simulink model "Copy_of_model_test"  (R2018b)
settings: Solver=ode5  StartTime=0.0  StopTime=10.0  FixedStep=0.01  RelTol=1e-3
values from neighbouring files (symbols this model uses):
  g = 9.81    [equations.m]    (also in general.m; general_lqi.m)
  m = 0.06    [equations.m]    (also in general.m = 0.057; general_lqi.m = 0.057)
  R = 1    [evaluateL.m]    (also in general.m = 4; general_lqi.m = 4)
  u_0 = R*x3_0    [general.m]    (also in general_lqi.m)
  x1_0 = 0.005    [general.m]    (also in general_lqi.m = 0.01)
  x2_0 = 0    [general.m]    (also in general_lqi.m)
  x3_0 = sqrt((-2*m*g)/first(x1_0))    [general.m]    (also in general_lqi.m)
  x_0 = [x1_0 x2_0 x3_0]    [general.m]    (also in general_lqi.m)
undefined symbols (not defined in the file or in its folder): K
settings Model: Creator=Kinga  LastModifiedBy=Kinga

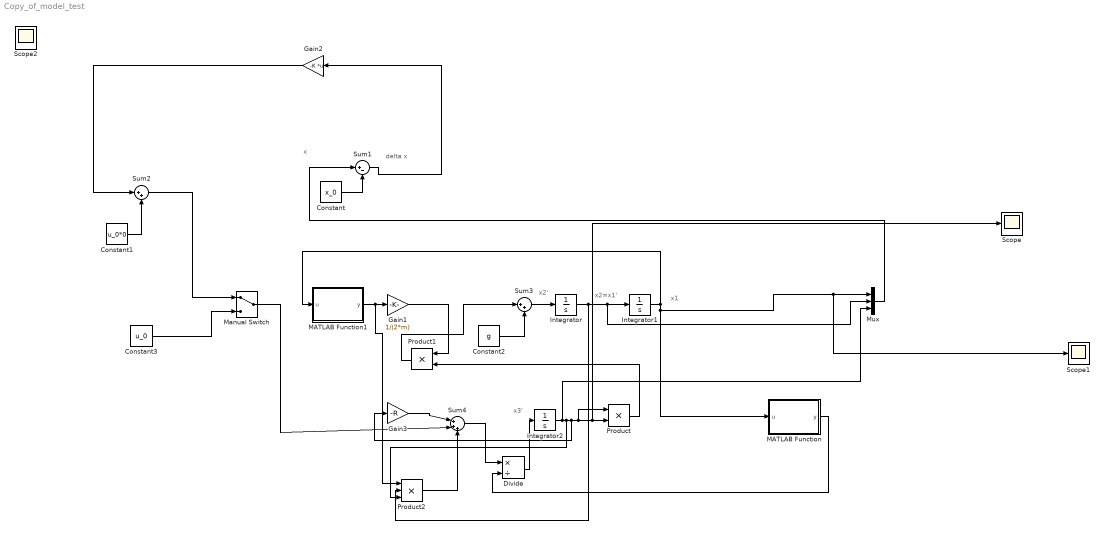
== system Copy_of_model_test ==
  note: x3'
  note: x1
  note: x2=x1'
  note: x2'
  note: delta x
  note: x
  Constant : Constant  Value=x_0
  Constant1 : Constant  Value=u_0*0
  Constant2 : Constant  Value=g
  Constant3 : Constant  Value=u_0
  Divide : Product  Inputs=*/
  Gain1 : Gain  Gain=1/(2*m)
  Gain2 : Gain  Gain=-K  Multiplication=Matrix(K*u) (u vector)
  Gain3 : Gain  Gain=-R
  Integrator : Integrator  InitialCondition=x2_0
  Integrator1 : Integrator  InitialCondition=x1_0
  Integrator2 : Integrator  InitialCondition=x3_0
  MATLAB Function : MATLAB Function  TreatAsAtomicUnit=on
  MATLAB Function1 : MATLAB Function  TreatAsAtomicUnit=on
  Manual Switch : ManualSwitch
  Mux : Mux  Inputs=3
  Product : Product
  Product1 : Product
  Product2 : Product  Inputs=3
  Scope : Scope
  Scope1 : Scope
  Sum1 : Sum  Inputs=|+-
  Sum2 : Sum  Inputs=|++
  Sum3 : Sum  Inputs=|++
  Sum4 : Sum  Inputs=|+++
  Scope2 : Scope
  wires:
  Constant/1 -> Sum1/2
  Sum1/1 -> Gain2/1
  Constant1/1 -> Sum2/2
  Gain2/1 -> Sum2/1
  Sum3/1 -> Integrator/1
  Constant2/1 -> Sum3/2
  Integrator/1 -> Product2/2, Mux/2, Integrator1/1
  MATLAB Function1/1(y) -> Product2/1, Gain1/1
  Integrator1/1 -> Scope1/1, Mux/1, MATLAB Function/1(u), MATLAB Function1/1(u)
  Product/1 -> Product1/2
  Gain1/1 -> Product1/1
  Product1/1 -> Sum3/1
  Gain3/1 -> Sum4/1
  Sum4/1 -> Divide/1
  MATLAB Function/1(y) -> Divide/2
  Divide/1 -> Integrator2/1
  Mux/1 -> Sum1/1
  Product2/1 -> Sum4/3
  Integrator2/1 -> Mux/3, Product2/3, Gain3/1, Product/1, Scope/1, Product/2
  Constant3/1 -> Manual Switch/2
  Manual Switch/1 -> Sum4/2
  Sum2/1 -> Manual Switch/1

== matlab function Copy_of_model_test/MATLAB Function1 ==
  data: u input; y output
function y = first(u)

a = 0.1017;
b = 0.01801;
c = -158.7;

y = c*b*exp(c*u);

== matlab function Copy_of_model_test/MATLAB Function ==
  data: u input; y output
function y = base(u)

a = 0.1017;
b = 0.01801;
c = -158.7;

y = a+b*exp(c*u);
